simulink model "Car_Control_6"  (R2021a)
settings: Solver=VariableStepAuto  StartTime=0.0  StopTime=180.0  RelTol=1e-3
libraries: fuzblock x1
settings Model: Creator=User  LastModifiedBy=User

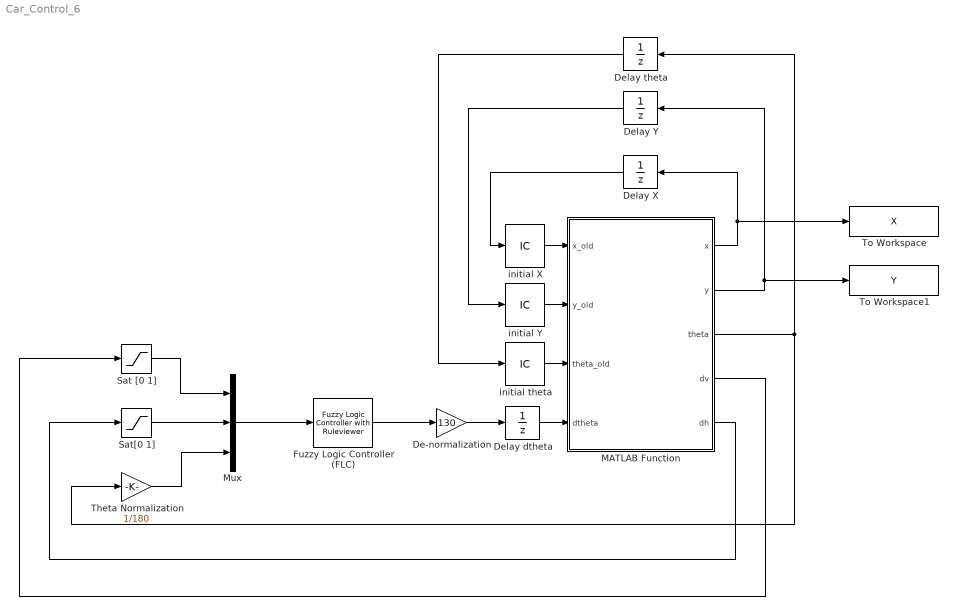
== system Car_Control_6 ==
  De-normalization : Gain  Gain=130
  Delay X : UnitDelay  SampleTime=0.1  HasFrameUpgradeWarning=on
  Delay Y : UnitDelay  SampleTime=0.1  HasFrameUpgradeWarning=on
  Delay dtheta : UnitDelay  SampleTime=0.1  HasFrameUpgradeWarning=on
  Delay theta : UnitDelay  SampleTime=0.1  HasFrameUpgradeWarning=on
  Fuzzy Logic Controller (FLC) : fuzblock/Fuzzy Logic  Controller  with Ruleviewer  fismatrix=FIS_Car  Ts=0.1
  MATLAB Function : MATLAB Function  TreatAsAtomicUnit=on
  Mux : Mux  Inputs=3
  Sat [0 1] : Saturate  UpperLimit=1  LowerLimit=0
  Sat[0 1] : Saturate  UpperLimit=1  LowerLimit=0
  Theta Normalization : Gain  Gain=1/180
  To Workspace : ToWorkspace  VariableName=X  SaveFormat=Timeseries  SampleTime=-1
  To Workspace1 : ToWorkspace  VariableName=Y  SaveFormat=Timeseries  SampleTime=-1
  initial X : InitialCondition  Value=3.2
  initial Y : InitialCondition  Value=0.5
  initial theta : InitialCondition  Value=0
  wires:
  MATLAB Function/3(theta) -> Delay theta/1, Theta Normalization/1
  Delay theta/1 -> initial theta/1
  MATLAB Function/2(y) -> To Workspace1/1, Delay Y/1
  Delay Y/1 -> initial Y/1
  MATLAB Function/1(x) -> To Workspace/1, Delay X/1
  Delay X/1 -> initial X/1
  Fuzzy Logic Controller (FLC)/1 -> De-normalization/1
  De-normalization/1 -> Delay dtheta/1
  Mux/1 -> Fuzzy Logic Controller (FLC)/1
  MATLAB Function/4(dv) -> Sat [0 1]/1
  MATLAB Function/5(dh) -> Sat[0 1]/1
  Theta Normalization/1 -> Mux/3
  initial X/1 -> MATLAB Function/1(x_old)
  initial Y/1 -> MATLAB Function/2(y_old)
  initial theta/1 -> MATLAB Function/3(theta_old)
  Sat[0 1]/1 -> Mux/2
  Sat [0 1]/1 -> Mux/1
  Delay dtheta/1 -> MATLAB Function/4(dtheta)

== matlab function Car_Control_6/MATLAB Function ==
  data: x output; x_old input; y output; y_old input; theta_old input; dtheta input; theta output; dv output; dh output
function [x, y, theta, dv, dh] = car_model(x_old, y_old, theta_old, dtheta)
    % Local variables
    if(x_old >= 10)
        u = 0;
    else
        u = 0.05;       % Constant car velocity 
    end
    
    t = 0.1;       % Delay between each calculation
    
    % Calculate the new angle of the car:
    theta = theta_old + dtheta;
    
    % Saturation for the new theta inside the [-180 180] 
    if(theta > 180)
        theta = 180;
    elseif(theta < -180)
       theta = -180;
    end
    
    % Calculation of the new position
    x = x_old + u*cos(theta/360*2*pi)*t;
    y = y_old + u*sin(theta/360*2*pi)*t;
    
    % Calculation of the horizontal distance from obstacle
    if (y <= 1)
        dh = 5 - x;
    elseif (y > 1 && y <= 2)
        dh = 6 - x;
    elseif (y > 2 && y <= 3)
        dh = 7 - x;
    else
        dh = 20 - x;
    end
    
    % Calculation of the vertical distance from obstacle
    if (x <= 5)
        dv = y;
    elseif (x > 5 && x <= 6)
        dv = y - 1;
    elseif (x > 6 && x <= 7)
        dv = y - 2;
    else
        dv = y - 3;
    end
end
